simulink model "VVVF_nt"  (R2018b)
settings: Solver=ode23tb  StartTime=0.0  StopTime=16  MaxStep=10e-6  RelTol=1e-4  EnableMultiTasking=on
libraries: powerlib x57
settings Model: SimulationMode=accelerator  Creator=Gong Linxiao  LastModifiedBy=vibra
settings DataIOCC: LimitDataPoints=on  SaveFormat=Array
settings OptimizationCC: LifeSpan=inf
settings DebuggingCC: SolverPrmCheckMsg=warning  SFUnexpectedBacktrackingDiag=warning  SFNoUnconditionalDefaultTransitionDiag=warning  SFExecutionAtInitializationDiag=none
settings HardwareCC: ProdBitPerPointer=32  ProdBitPerSizeT=32  ProdBitPerPtrDiffT=32  ProdLargestAtomicFloat=None  ProdIntDivRoundTo=Undefined  ProdEndianess=Unspecified  ProdWordSize=32  ProdHWDeviceType=32-bit Generic
settings ModelReferenceCC: PropagateSignalLabelsOutOfModel=off
settings SFSimCC: SimUseLocalCustomCode=off
settings RTWCC: RTWUseLocalCustomCode=off
settings CodeAppCC: StateflowObjectComments=on
settings GRTTargetCC: TargetLangStandard=C89/C90 (ANSI)  GeneratePreprocessorConditionals=Disable all
settings ConfigComp: CovMetricSettings=dw  CovHtmlReporting=on  CovSaveCumulativeToWorkspaceVar=on  CovSaveSingleToWorkspaceVar=on  CovExternalEMLEnable=off  CovSFcnEnable=off
settings SimscapeCC: SimscapeNormalizeSystem=off

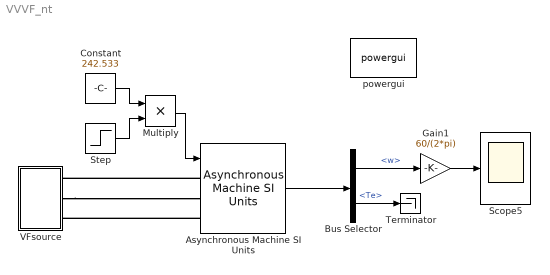
== system VVVF_nt ==
  Asynchronous Machine SI Units : powerlib/Machines/Asynchronous Machine SI Units  RotorType=Squirrel-cage  PresetModel="18:  50 HP (37KW)   400 V 50Hz 1480 RPM"  MechanicalLoad=Torque Tm  ShowDetailedParameters=on  ReferenceFrame=Stationary  Units=SI  MeasurementBus=on  NominalParameters=[3.7e+04 400 50]  Stator=[0.08233 0.000724]  Rotor=[0.0503 0.000724]  Cage1=[ 0.022 0.226/377]  Cage2=[ 0.022 0.226/377]  Lm=0.02711  Mechanical=[0.37 0.02791 2]  PolePairs=2  InitialConditions=[1 0 0 0 0 0 0 0]  SimulateSaturation=off  Saturation=[14.03593122, 27.81365428, 53.79336849, 72.68890987, 97.98006896, 148.6815601, 215.7428561, 302.9841135, 420.4778367 ; 230, 322, 414, 460, 506, 552, 598, 644, 690]  LoadFlowParameters=1492000  TsPowergui=0  TsBlock=-1  IterativeModel=Trapezoidal non iterative  IterativeDiscreteModel=Trapezoidal non iterative  Pmec=0
      settings: SourceProductName=Simscape Electrical
  Bus Selector : BusSelector  OutputSignals=w,Te
  Constant : Constant  Value=242.533  SampleTime=Inf
  Gain1 : Gain  Gain=60/(2*pi)
  Multiply : Product
  Scope5 : Scope
  Step : Step  SampleTime=0
  Terminator : Terminator
  VFsource : Subsystem
  powergui : powerlib/powergui  Priority=1  SimulationMode=Continuous  SampleTime=50e-6  frequency=60  Iterations=50  frequencyindice=50  Pbase=100e6  ErrMax=1e-4  UnitsV=kV  UnitsW=MW  buscounter=0  FunctionMessages=off  echomessages=off  EnableUseOfTLC=off  CurrentSourceSwitches=on  DisableSnubberDevices=off  DisableRonSwitches=off  DisableVfSwitches=off  DisplayEquations=off  SolverType=Tustin  Interpol=off  ExternalGateDelay=off  methode=off  Ts=0  x0status=blocks  SPID=off  SwTol=0  HookPort=off  RestoreLinks=warning  ResistiveCurrentMeasurement=off  Frange=[0:2:500]  Ylog=off  Xlog=on  ShowGrid=off  save=off  variable=ZData  structure=0  ZoomFFT=off  StartTime=0.0  cycles=1  DisplayStyle=1  fundamental=60  FreqAxis=off  MaxFrequency=1000  frequencyindicesteady=1  RmsSteady=2  display=off
  wires:
  Asynchronous Machine SI Units/1 -> Bus Selector/1
  Bus Selector/1 -> Gain1/1  "<w>"
  Gain1/1 -> Scope5/1
  Step/1 -> Multiply/2
  Constant/1 -> Multiply/1
  Multiply/1 -> Asynchronous Machine SI Units/1
  Bus Selector/2 -> Terminator/1  "<Te>"
  connections:
  Asynchronous Machine SI Units/LConn3 -- VFsource/RConn3
  Asynchronous Machine SI Units/LConn1 -- VFsource/RConn1
  VFsource/RConn2 -- Asynchronous Machine SI Units/LConn2

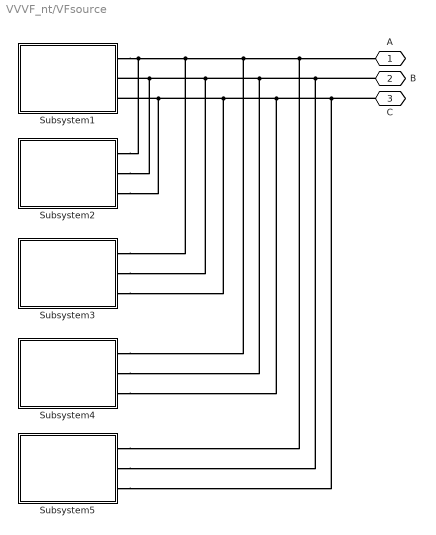
== system VVVF_nt/VFsource ==
  Subsystem1 : Subsystem
  Subsystem2 : Subsystem
  Subsystem3 : Subsystem
  Subsystem4 : Subsystem
  Subsystem5 : Subsystem
  A : PMIOPort  Side=Right
  B : PMIOPort  Port=2  Side=Right
  C : PMIOPort  Port=3  Side=Right
  connections:
  C/RConn1 -- Subsystem5/LConn3 -- Subsystem4/LConn3 -- Subsystem3/LConn3 -- Subsystem2/LConn3 -- Subsystem1/LConn3
  B/RConn1 -- Subsystem5/LConn2 -- Subsystem4/LConn2 -- Subsystem3/LConn2 -- Subsystem2/LConn2 -- Subsystem1/LConn2
  Subsystem1/LConn1 -- Subsystem2/LConn1 -- Subsystem3/LConn1 -- Subsystem4/LConn1 -- Subsystem5/LConn1 -- A/RConn1

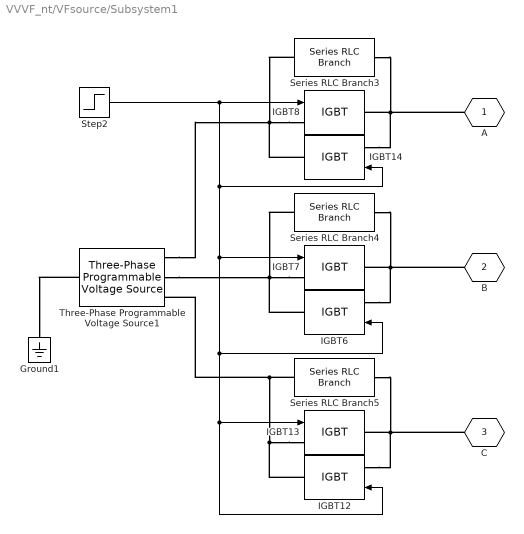
== system VVVF_nt/VFsource/Subsystem1 ==
  Ground1 : powerlib/Elements/Ground  LConnTagsString=a
      settings: SourceProductName=Simscape Electrical
  IGBT{6..8,12..14} (6 alike) : powerlib/Power Electronics/IGBT  Ron=1e-5  Lon=0  Vf=1  Tf=1e-6  Tt=2e-6  IC=0  Rs=inf  Cs=inf  Measurements=off
  Series RLC Branch3 : powerlib/Elements/Series RLC Branch  LConnTagsString=__new0  RConnTagsString=__new0  BranchType=R  Resistance=1e6  Inductance=1e-3  SetiL0=off  InitialCurrent=0  Capacitance=1e-6  Setx0=off  InitialVoltage=0  Measurements=None
  Series RLC Branch4 : powerlib/Elements/Series RLC Branch  LConnTagsString=__new0  RConnTagsString=__new0  BranchType=R  Resistance=1e6  Inductance=1e-3  SetiL0=off  InitialCurrent=0  Capacitance=1e-6  Setx0=off  InitialVoltage=0  Measurements=None
  Series RLC Branch5 : powerlib/Elements/Series RLC Branch  LConnTagsString=__new0  RConnTagsString=__new0  BranchType=R  Resistance=1e6  Inductance=1e-3  SetiL0=off  InitialCurrent=0  Capacitance=1e-6  Setx0=off  InitialVoltage=0  Measurements=None
  Step2 : Step  Time=2  Before=1  After=0  SampleTime=0
  Three-Phase Programmable Voltage Source1 : powerlib/Electrical Sources/Three-Phase Programmable Voltage Source  PositiveSequence=[400 0 50]  VariationEntity=None  VariationType=Table of time-amplitude pairs  VariationTypeAlt=Step  VariationStep=20  VariationRate=30  VariationMagnitude=0.3  VariationFrequency=2  VariationTiming=[1 5]  VariationPhaseA=off  Amplitudes=[1 0.8 1.2 1.0]  TimeValues=[0 0.1 0.15 0.2]  HarmonicGeneration=off  HarmonicA=[3 0.2 -25 0]  HarmonicB=[2 0.15 35 2]  Timing="[0.05  3]"  BusType=PV  Pref=0  Qref=0  Qmin=-inf  Qmax=inf
      settings: SourceProductName=Simscape Electrical
  A : PMIOPort  Tag=PMCPort  Side=Left
  B : PMIOPort  Tag=PMCPort  Port=2  Side=Left
  C : PMIOPort  Tag=PMCPort  Port=3  Side=Left
  wires:
  Step2/1 -> IGBT13/1, IGBT12/1, IGBT6/1, IGBT7/1, IGBT14/1, IGBT8/1
  connections:
  IGBT14/LConn1 -- Series RLC Branch3/RConn1 -- IGBT8/RConn1 -- A/RConn1
  IGBT13/LConn1 -- IGBT12/RConn1 -- Series RLC Branch5/LConn1 -- Three-Phase Programmable Voltage Source1/RConn3
  IGBT7/LConn1 -- IGBT6/RConn1 -- Series RLC Branch4/LConn1 -- Three-Phase Programmable Voltage Source1/RConn2
  IGBT12/LConn1 -- Series RLC Branch5/RConn1 -- IGBT13/RConn1 -- C/RConn1
  IGBT6/LConn1 -- Series RLC Branch4/RConn1 -- IGBT7/RConn1 -- B/RConn1
  IGBT8/LConn1 -- IGBT14/RConn1 -- Three-Phase Programmable Voltage Source1/RConn1 -- Series RLC Branch3/LConn1
  Three-Phase Programmable Voltage Source1/LConn1 -- Ground1/LConn1

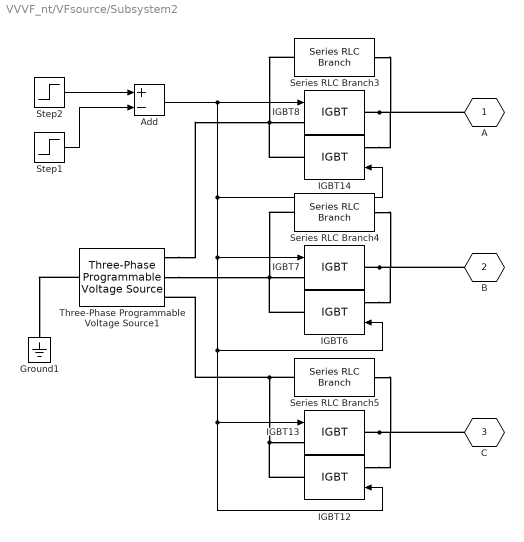
== system VVVF_nt/VFsource/Subsystem2 ==
  Add : Sum  Inputs=+-
  Ground1 : powerlib/Elements/Ground  LConnTagsString=a
      settings: SourceProductName=Simscape Electrical
  IGBT{6..8,12..14} (6 alike) : powerlib/Power Electronics/IGBT  Ron=1e-5  Lon=0  Vf=1  Tf=1e-6  Tt=2e-6  IC=0  Rs=inf  Cs=inf  Measurements=off
  Series RLC Branch3 : powerlib/Elements/Series RLC Branch  LConnTagsString=__new0  RConnTagsString=__new0  BranchType=R  Resistance=1e6  Inductance=1e-3  SetiL0=off  InitialCurrent=0  Capacitance=1e-6  Setx0=off  InitialVoltage=0  Measurements=None
  Series RLC Branch4 : powerlib/Elements/Series RLC Branch  LConnTagsString=__new0  RConnTagsString=__new0  BranchType=R  Resistance=1e6  Inductance=1e-3  SetiL0=off  InitialCurrent=0  Capacitance=1e-6  Setx0=off  InitialVoltage=0  Measurements=None
  Series RLC Branch5 : powerlib/Elements/Series RLC Branch  LConnTagsString=__new0  RConnTagsString=__new0  BranchType=R  Resistance=1e6  Inductance=1e-3  SetiL0=off  InitialCurrent=0  Capacitance=1e-6  Setx0=off  InitialVoltage=0  Measurements=None
  Step1 : Step  Time=4  SampleTime=0
  Step2 : Step  Time=2  SampleTime=0
  Three-Phase Programmable Voltage Source1 : powerlib/Electrical Sources/Three-Phase Programmable Voltage Source  PositiveSequence="[320  0 40]"  VariationEntity=None  VariationType=Table of time-amplitude pairs  VariationTypeAlt=Step  VariationStep=20  VariationRate=30  VariationMagnitude=0.3  VariationFrequency=2  VariationTiming=[1 5]  VariationPhaseA=off  Amplitudes=[1 0.8 1.2 1.0]  TimeValues=[0 0.1 0.15 0.2]  HarmonicGeneration=off  HarmonicA=[3 0.2 -25 0]  HarmonicB=[2 0.15 35 2]  Timing="[0.05  3]"  BusType=PV  Pref=0  Qref=0  Qmin=-inf  Qmax=inf
      settings: SourceProductName=Simscape Electrical
  A : PMIOPort  Tag=PMCPort  Side=Left
  B : PMIOPort  Tag=PMCPort  Port=2  Side=Left
  C : PMIOPort  Tag=PMCPort  Port=3  Side=Left
  wires:
  Step2/1 -> Add/1
  Step1/1 -> Add/2
  Add/1 -> IGBT8/1, IGBT7/1, IGBT13/1, IGBT12/1, IGBT6/1, IGBT14/1
  connections:
  IGBT8/RConn1 -- A/RConn1 -- IGBT14/LConn1 -- Series RLC Branch3/RConn1
  Series RLC Branch5/LConn1 -- IGBT13/LConn1 -- IGBT12/RConn1 -- Three-Phase Programmable Voltage Source1/RConn3
  Series RLC Branch4/LConn1 -- Three-Phase Programmable Voltage Source1/RConn2 -- IGBT7/LConn1 -- IGBT6/RConn1
  IGBT13/RConn1 -- C/RConn1 -- IGBT12/LConn1 -- Series RLC Branch5/RConn1
  IGBT7/RConn1 -- B/RConn1 -- IGBT6/LConn1 -- Series RLC Branch4/RConn1
  Three-Phase Programmable Voltage Source1/RConn1 -- IGBT8/LConn1 -- IGBT14/RConn1 -- Series RLC Branch3/LConn1
  Three-Phase Programmable Voltage Source1/LConn1 -- Ground1/LConn1

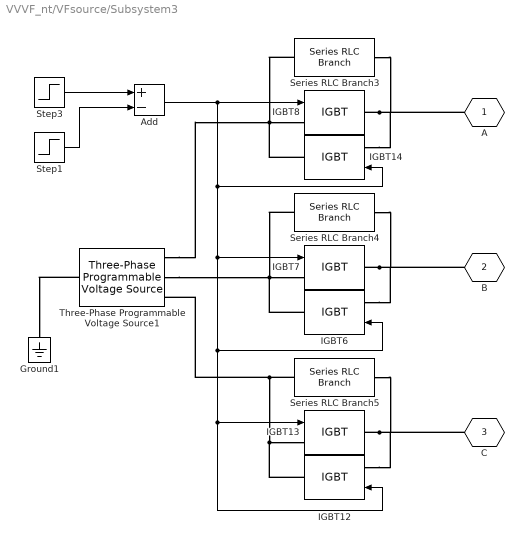
== system VVVF_nt/VFsource/Subsystem3 ==
  Add : Sum  Inputs=+-
  Ground1 : powerlib/Elements/Ground  LConnTagsString=a
      settings: SourceProductName=Simscape Electrical
  IGBT{6..8,12..14} (6 alike) : powerlib/Power Electronics/IGBT  Ron=1e-5  Lon=0  Vf=1  Tf=1e-6  Tt=2e-6  IC=0  Rs=inf  Cs=inf  Measurements=off
  Series RLC Branch3 : powerlib/Elements/Series RLC Branch  LConnTagsString=__new0  RConnTagsString=__new0  BranchType=R  Resistance=1e6  Inductance=1e-3  SetiL0=off  InitialCurrent=0  Capacitance=1e-6  Setx0=off  InitialVoltage=0  Measurements=None
  Series RLC Branch4 : powerlib/Elements/Series RLC Branch  LConnTagsString=__new0  RConnTagsString=__new0  BranchType=R  Resistance=1e6  Inductance=1e-3  SetiL0=off  InitialCurrent=0  Capacitance=1e-6  Setx0=off  InitialVoltage=0  Measurements=None
  Series RLC Branch5 : powerlib/Elements/Series RLC Branch  LConnTagsString=__new0  RConnTagsString=__new0  BranchType=R  Resistance=1e6  Inductance=1e-3  SetiL0=off  InitialCurrent=0  Capacitance=1e-6  Setx0=off  InitialVoltage=0  Measurements=None
  Step1 : Step  Time=7  SampleTime=0
  Step3 : Step  Time=4  SampleTime=0
  Three-Phase Programmable Voltage Source1 : powerlib/Electrical Sources/Three-Phase Programmable Voltage Source  PositiveSequence="[240  0 30]"  VariationEntity=None  VariationType=Table of time-amplitude pairs  VariationTypeAlt=Step  VariationStep=20  VariationRate=30  VariationMagnitude=0.3  VariationFrequency=2  VariationTiming=[1 5]  VariationPhaseA=off  Amplitudes=[1 0.8 1.2 1.0]  TimeValues=[0 0.1 0.15 0.2]  HarmonicGeneration=off  HarmonicA=[3 0.2 -25 0]  HarmonicB=[2 0.15 35 2]  Timing="[0.05  3]"  BusType=PV  Pref=0  Qref=0  Qmin=-inf  Qmax=inf
      settings: SourceProductName=Simscape Electrical
  A : PMIOPort  Tag=PMCPort  Side=Left
  B : PMIOPort  Tag=PMCPort  Port=2  Side=Left
  C : PMIOPort  Tag=PMCPort  Port=3  Side=Left
  wires:
  Step1/1 -> Add/2
  Step3/1 -> Add/1
  Add/1 -> IGBT8/1, IGBT7/1, IGBT6/1, IGBT12/1, IGBT13/1, IGBT14/1
  connections:
  IGBT8/RConn1 -- A/RConn1 -- IGBT14/LConn1 -- Series RLC Branch3/RConn1
  Series RLC Branch5/LConn1 -- IGBT13/LConn1 -- IGBT12/RConn1 -- Three-Phase Programmable Voltage Source1/RConn3
  Series RLC Branch4/LConn1 -- Three-Phase Programmable Voltage Source1/RConn2 -- IGBT7/LConn1 -- IGBT6/RConn1
  IGBT13/RConn1 -- C/RConn1 -- IGBT12/LConn1 -- Series RLC Branch5/RConn1
  IGBT7/RConn1 -- B/RConn1 -- IGBT6/LConn1 -- Series RLC Branch4/RConn1
  Three-Phase Programmable Voltage Source1/RConn1 -- IGBT8/LConn1 -- IGBT14/RConn1 -- Series RLC Branch3/LConn1
  Three-Phase Programmable Voltage Source1/LConn1 -- Ground1/LConn1

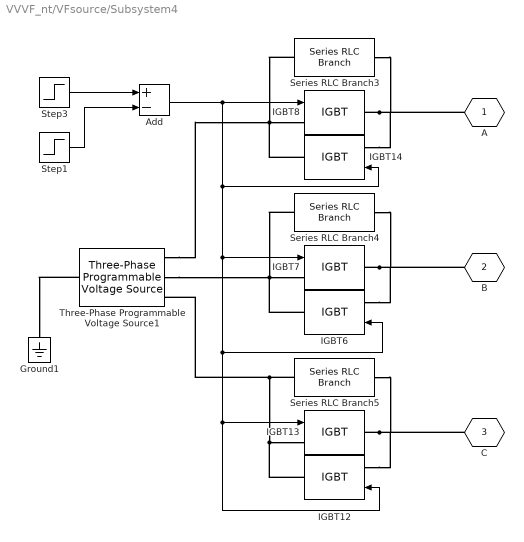
== system VVVF_nt/VFsource/Subsystem4 ==
  Add : Sum  Inputs=+-
  Ground1 : powerlib/Elements/Ground  LConnTagsString=a
      settings: SourceProductName=Simscape Electrical
  IGBT{6..8,12..14} (6 alike) : powerlib/Power Electronics/IGBT  Ron=1e-5  Lon=0  Vf=1  Tf=1e-6  Tt=2e-6  IC=0  Rs=inf  Cs=inf  Measurements=off
  Series RLC Branch3 : powerlib/Elements/Series RLC Branch  LConnTagsString=__new0  RConnTagsString=__new0  BranchType=R  Resistance=1e6  Inductance=1e-3  SetiL0=off  InitialCurrent=0  Capacitance=1e-6  Setx0=off  InitialVoltage=0  Measurements=None
  Series RLC Branch4 : powerlib/Elements/Series RLC Branch  LConnTagsString=__new0  RConnTagsString=__new0  BranchType=R  Resistance=1e6  Inductance=1e-3  SetiL0=off  InitialCurrent=0  Capacitance=1e-6  Setx0=off  InitialVoltage=0  Measurements=None
  Series RLC Branch5 : powerlib/Elements/Series RLC Branch  LConnTagsString=__new0  RConnTagsString=__new0  BranchType=R  Resistance=1e6  Inductance=1e-3  SetiL0=off  InitialCurrent=0  Capacitance=1e-6  Setx0=off  InitialVoltage=0  Measurements=None
  Step1 : Step  Time=12  SampleTime=0
  Step3 : Step  Time=7  SampleTime=0
  Three-Phase Programmable Voltage Source1 : powerlib/Electrical Sources/Three-Phase Programmable Voltage Source  PositiveSequence=[160 0 20]  VariationEntity=None  VariationType=Table of time-amplitude pairs  VariationTypeAlt=Step  VariationStep=20  VariationRate=30  VariationMagnitude=0.3  VariationFrequency=2  VariationTiming=[1 5]  VariationPhaseA=off  Amplitudes=[1 0.8 1.2 1.0]  TimeValues=[0 0.1 0.15 0.2]  HarmonicGeneration=off  HarmonicA=[3 0.2 -25 0]  HarmonicB=[2 0.15 35 2]  Timing="[0.05  3]"  BusType=PV  Pref=0  Qref=0  Qmin=-inf  Qmax=inf
      settings: SourceProductName=Simscape Electrical
  A : PMIOPort  Tag=PMCPort  Side=Left
  B : PMIOPort  Tag=PMCPort  Port=2  Side=Left
  C : PMIOPort  Tag=PMCPort  Port=3  Side=Left
  wires:
  Step3/1 -> Add/1
  Step1/1 -> Add/2
  Add/1 -> IGBT8/1, IGBT14/1, IGBT7/1, IGBT12/1, IGBT13/1, IGBT6/1
  connections:
  IGBT8/RConn1 -- A/RConn1 -- IGBT14/LConn1 -- Series RLC Branch3/RConn1
  Series RLC Branch5/LConn1 -- IGBT13/LConn1 -- IGBT12/RConn1 -- Three-Phase Programmable Voltage Source1/RConn3
  Series RLC Branch4/LConn1 -- Three-Phase Programmable Voltage Source1/RConn2 -- IGBT7/LConn1 -- IGBT6/RConn1
  IGBT13/RConn1 -- C/RConn1 -- IGBT12/LConn1 -- Series RLC Branch5/RConn1
  IGBT7/RConn1 -- B/RConn1 -- IGBT6/LConn1 -- Series RLC Branch4/RConn1
  Three-Phase Programmable Voltage Source1/RConn1 -- IGBT8/LConn1 -- IGBT14/RConn1 -- Series RLC Branch3/LConn1
  Three-Phase Programmable Voltage Source1/LConn1 -- Ground1/LConn1

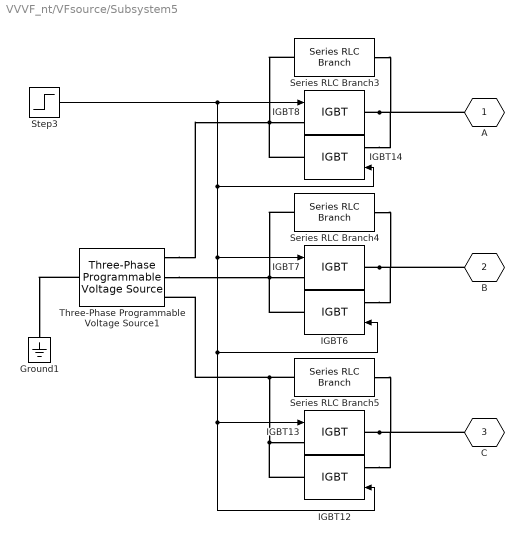
== system VVVF_nt/VFsource/Subsystem5 ==
  Ground1 : powerlib/Elements/Ground  LConnTagsString=a
      settings: SourceProductName=Simscape Electrical
  IGBT{6..8,12..14} (6 alike) : powerlib/Power Electronics/IGBT  Ron=1e-5  Lon=0  Vf=1  Tf=1e-6  Tt=2e-6  IC=0  Rs=inf  Cs=inf  Measurements=off
  Series RLC Branch3 : powerlib/Elements/Series RLC Branch  LConnTagsString=__new0  RConnTagsString=__new0  BranchType=R  Resistance=1e6  Inductance=1e-3  SetiL0=off  InitialCurrent=0  Capacitance=1e-6  Setx0=off  InitialVoltage=0  Measurements=None
  Series RLC Branch4 : powerlib/Elements/Series RLC Branch  LConnTagsString=__new0  RConnTagsString=__new0  BranchType=R  Resistance=1e6  Inductance=1e-3  SetiL0=off  InitialCurrent=0  Capacitance=1e-6  Setx0=off  InitialVoltage=0  Measurements=None
  Series RLC Branch5 : powerlib/Elements/Series RLC Branch  LConnTagsString=__new0  RConnTagsString=__new0  BranchType=R  Resistance=1e6  Inductance=1e-3  SetiL0=off  InitialCurrent=0  Capacitance=1e-6  Setx0=off  InitialVoltage=0  Measurements=None
  Step3 : Step  Time=12  SampleTime=0
  Three-Phase Programmable Voltage Source1 : powerlib/Electrical Sources/Three-Phase Programmable Voltage Source  PositiveSequence=[80 0 10]  VariationEntity=None  VariationType=Table of time-amplitude pairs  VariationTypeAlt=Step  VariationStep=20  VariationRate=30  VariationMagnitude=0.3  VariationFrequency=2  VariationTiming=[1 5]  VariationPhaseA=off  Amplitudes=[1 0.8 1.2 1.0]  TimeValues=[0 0.1 0.15 0.2]  HarmonicGeneration=off  HarmonicA=[3 0.2 -25 0]  HarmonicB=[2 0.15 35 2]  Timing="[0.05  3]"  BusType=PV  Pref=0  Qref=0  Qmin=-inf  Qmax=inf
      settings: SourceProductName=Simscape Electrical
  A : PMIOPort  Tag=PMCPort  Side=Left
  B : PMIOPort  Tag=PMCPort  Port=2  Side=Left
  C : PMIOPort  Tag=PMCPort  Port=3  Side=Left
  wires:
  Step3/1 -> IGBT8/1, IGBT14/1, IGBT7/1, IGBT6/1, IGBT13/1, IGBT12/1
  connections:
  IGBT8/RConn1 -- A/RConn1 -- IGBT14/LConn1 -- Series RLC Branch3/RConn1
  Series RLC Branch5/LConn1 -- IGBT13/LConn1 -- IGBT12/RConn1 -- Three-Phase Programmable Voltage Source1/RConn3
  Series RLC Branch4/LConn1 -- Three-Phase Programmable Voltage Source1/RConn2 -- IGBT7/LConn1 -- IGBT6/RConn1
  IGBT13/RConn1 -- C/RConn1 -- IGBT12/LConn1 -- Series RLC Branch5/RConn1
  IGBT7/RConn1 -- B/RConn1 -- IGBT6/LConn1 -- Series RLC Branch4/RConn1
  Three-Phase Programmable Voltage Source1/RConn1 -- IGBT8/LConn1 -- IGBT14/RConn1 -- Series RLC Branch3/LConn1
  Three-Phase Programmable Voltage Source1/LConn1 -- Ground1/LConn1
